simulink model "NeuromuscularModel"  (R2019b)
settings: Solver=ode15s  StartTime=0.0  StopTime=inf  MaxStep=.01  RelTol=1e-4  AbsTol=1e-6  EnableMultiTasking=on
values from neighbouring files (symbols this model uses):
  LceOffsetTA = 1-0.5*w    [ControlParams2.m]
  legLengthClr = .9    (= 0.9)    [ControlParams2.m]    (also in assignGains.m = Gains(20); assignGains2.m = Gains(20); assignGainsSagittal.m = GainsSagittal(39))
  LongDelay = 0.020    (= 0.02)    [ControlParams2.m]
  MidDelay = 0.010    (= 0.01)    [ControlParams2.m]
  N = 82    [vcmaes_1.5cm_0.9ms_Umb10_kneelim1_mstoptorque2.mat]
  ShortDelay = 0.005    [ControlParams2.m]
  simbiconGainD = 5*pi/180    (= 0.0872664625997)    [ControlParams2.m]    (also in assignGains.m = Gains(21); assignGains2.m = Gains(21); assignGainsSagittal.m = GainsSagittal(41))
  simbiconGainDAbd = 0.1421    [ControlParams2.m]    (also in assignGains.m = Gains(33))
  simbiconGainV = 5*pi/180    (= 0.0872664625997)    [ControlParams2.m]    (also in assignGains.m = Gains(22); assignGains2.m = Gains(22); assignGainsSagittal.m = GainsSagittal(42))
  simbiconGainVAbd = 0.2148    [ControlParams2.m]    (also in assignGains.m = Gains(34))
  simbiconLegAngle0 = 85*pi/180    (= 1.4835298642)    [ControlParams2.m]    (also in assignGains.m = Gains(23); assignGains2.m = Gains(23); assignGainsSagittal.m = GainsSagittal(40))
  simbiconLegAngle0Abd = -0.0133    [ControlParams2.m]    (also in assignGains.m = Gains(32))
undefined symbols (not defined in the file or in its folder): footCenterToCGDist, footInertia, footMass, g, hatHipToCenterDistLen, loptGAS, loptTA, lslackGAS, magnitude, phimaxGASa, phimaxGASk, phirefGASa, phirefGASk, rGASa, rGASk, rhoGASa, rhoGASk, X, Y, Z
libraries: NeuroMuscularLibrary x101, nesl_utility x30, sm_lib x21, simulink x4, simulink_extras x2, NeuroMuscularLibrary2 x2
(part 1 of 3)
settings Model: SimulationMode=rapid-accelerator  ParamWorkspaceSource=ReferencedWorkspace  ExtModeTrigDuration=100  TunableVars=GainGAS,GainGLU,GainHAM,GainKneeOverExt,GainSOL,GainSOLTA,GainTA,GainVAS,Kglu,PosGainGG,SpeedGainGG,groundTheta,groundX,groundZ,hipDGain,hipPGain,kneeExtendGain,kneeFlexGain,kneeHoldGain1,kneeHoldGain2,kneeStopGain,legAngleFilter,legLengthClr,simbiconGainD,simbiconGainV,simbiconLegAngle0  TunableVarsStorageClass=Auto,Auto,Auto,Auto,Auto,Auto,Auto,Auto,Auto,Auto,Auto,Auto,Auto,Auto,Auto,Auto,Auto,Auto,Auto,Auto,Auto,Auto,Auto,Auto,Auto,Auto  TunableVarsTypeQualifier=,,,,,,,,,,,,,,,,,,,,,,,,,  Creator=nitisht  LastModifiedBy=Nathan
settings SolverCC: AutoScaleAbsTol=off  ZeroCrossAlgorithm=Adaptive
settings DataIOCC: LimitDataPoints=on  SaveFinalState=on  SaveFormat=StructureWithTime  SaveOutput=off  SaveState=on  ReturnWorkspaceOutputs=off  StateSaveName=tmp_raccel_xout  SignalLoggingName=tmp_raccel_logsout
settings OptimizationCC: DefaultParameterBehavior=Inlined  EfficientMapNaN2IntZero=off  LifeSpan=inf  SimCompilerOptimization=on  AccelVerboseBuild=on
settings DebuggingCC: SaveWithDisabledLinksMsg=none  UnderspecifiedInitializationDetection=Classic  MergeDetectMultiDrivingBlocksExec=none  IgnoredZcDiagnostic=none  SolverPrmCheckMsg=warning  StateNameClashWarn=warning  SFUnexpectedBacktrackingDiag=warning  SFNoUnconditionalDefaultTransitionDiag=warning  SFExecutionAtInitializationDiag=none  ArithmeticOperatorsInVariantConditions=warning
settings HardwareCC: ProdBitPerPointer=32  ProdBitPerSizeT=32  ProdBitPerPtrDiffT=32  ProdLargestAtomicFloat=None  ProdIntDivRoundTo=Undefined  ProdEndianess=Unspecified  ProdWordSize=32  ProdHWDeviceType=Generic->Unspecified (assume 32-bit Generic)  TargetBitPerPointer=64  TargetBitPerSizeT=64  TargetBitPerPtrDiffT=64  TargetLongLongMode=on  TargetIntDivRoundTo=Zero  TargetEndianess=LittleEndian  TargetWordSize=64  TargetHWDeviceType=MATLAB Host  ProdEqTarget=off
settings ModelReferenceCC: PropagateSignalLabelsOutOfModel=off
settings SFSimCC: SFSimEcho=off  SimUseLocalCustomCode=off  CustomCodeUndefinedFunction=UseInterfaceOnly
settings RTWCC: SystemTargetFile=raccel.tlc  TemplateMakefile=raccel_default_tmf  RTWUseLocalCustomCode=off  RTWUseSimCustomCode=on
settings CodeAppCC: GenerateComments=off  MaxIdLength=128  MangleLength=10  SimulinkBlockComments=off
settings RaccelTargetCC: GeneratePreprocessorConditionals=Disable all  MultiInstanceERTCode=off  PreserveStateflowLocalDataDimensions=off  ENABLE_SLEXEC_SSBRIDGE=0  RTWCAPIParams=off
settings ConfigComp: CovMetricSettings=dw  CovHtmlReporting=on  CovSaveCumulativeToWorkspaceVar=on  CovSaveSingleToWorkspaceVar=on  CovExternalEMLEnable=off  CovSFcnEnable=off
settings SimscapeCC: SimscapeNormalizeSystem=off
settings ConfigurationSet: Description=SimMechanics 2G

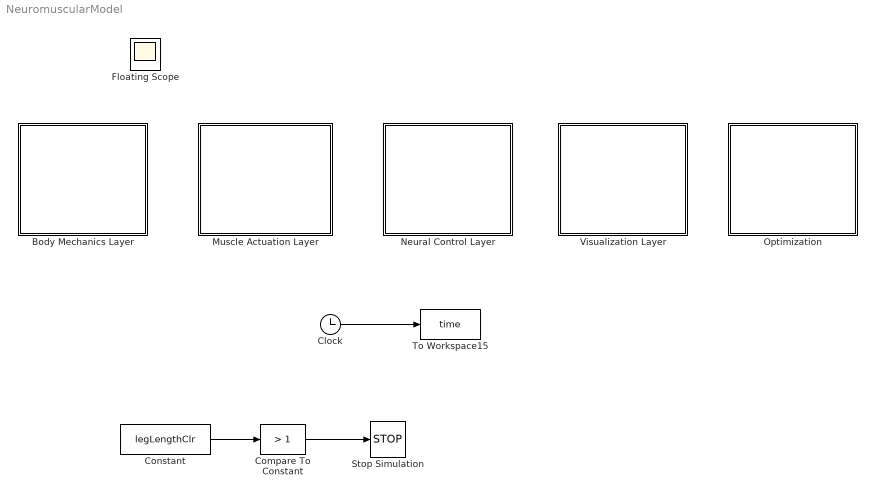
== system NeuromuscularModel ==
  Body Mechanics Layer : Subsystem
  Clock : Clock
  Compare To Constant : simulink/Logic and Bit Operations/Compare To Constant  relop=>  const=1  OutDataTypeStr=boolean
  Constant : Constant  Value=legLengthClr
  Muscle Actuation Layer : Subsystem
  Neural Control Layer : Subsystem
  Optimization : Subsystem
  Stop Simulation : Stop
  To Workspace15 : ToWorkspace  VariableName=time  SampleTime=-1
      settings: MaxDataPoints=1
  Visualization Layer : Subsystem
  Floating Scope : Scope
  wires:
  Clock/1 -> To Workspace15/1
  Compare To Constant/1 -> Stop Simulation/1
  Constant/1 -> Compare To Constant/1

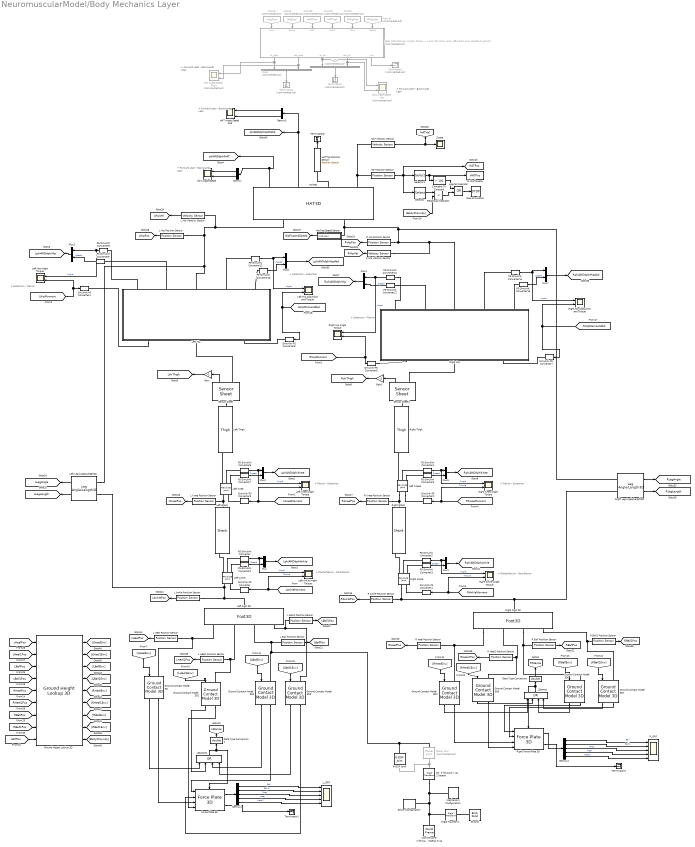
== system NeuromuscularModel/Body Mechanics Layer ==
  note: + Plantarflexion
      | -  Dorsiflexion
  note: + Flexion
      | -  Extension
  note: + Extension
      | -  Flexion
  note: + Forward Lean
      | -  Backwards Lean
  note: + Extension
      | -  Flexion
  note: + Plantarflexion
      | -  Dorsiflexion
  note: + Flexion
      | -  Extension
  note: + Forward Lean
      | -  Backwards Lean
  note: + Abduction
      | -  Adduction
  note: + Forward Lean
      | -  Backwards Lean
  note: + Forward Lean
      | -  Backwards Lean
  6-DOF Joint : sm_lib/Joints/6-DOF Joint  JointMode=Normal  SenseConstraintForce=off  SenseConstraintForceX=off  SenseConstraintForceY=off  SenseConstraintForceZ=off  SenseConstraintTorque=off  SenseConstraintTorqueX=off  SenseConstraintTorqueY=off  SenseConstraintTorqueZ=off  SenseTotalForce=off  SenseTotalForceX=off  SenseTotalForceY=off  SenseTotalForceZ=off  SenseTotalTorque=off  SenseTotalTorqueX=off  SenseTotalTorqueY=off  SenseTotalTorqueZ=off  CompositeWrenchDir=FollowerOnBase  CompositeWrenchFrame=BaseFrame  PxEquilibriumPosition=0  PxEquilibriumPositionUnits=m  PxSpringStiffness=0  PxSpringStiffnessUnits=N/m  PxDampingCoefficient=0  PxDampingCoefficientUnits=N/(m/s)  PxTorqueActuationMode=NoTorque  PxMotionActuationMode=ComputedMotion  PxSensePosition=off  PxSenseVelocity=off  PxSenseAcceleration=off  PxSenseTorqueForce=off  PxSenseLowerLimitTorqueForce=off  PxSenseUpperLimitTorqueForce=off  PxLowerLimitSpecify=off  PxLowerLimitBound=-1  PxLowerLimitBoundUnits=m  PxLowerLimitStiffness=1e6  PxLowerLimitStiffnessUnits=N/m  PxLowerLimitDamping=1e3  PxLowerLimitDampingUnits=N/(m/s)  PxLowerLimitTransitionRegionWidth=1e-4  PxLowerLimitTransitionRegionWidthUnits=m  PxUpperLimitSpecify=off  PxUpperLimitBound=1  PxUpperLimitBoundUnits=m  PxUpperLimitStiffness=1e6  PxUpperLimitStiffnessUnits=N/m  PxUpperLimitDamping=1e3  PxUpperLimitDampingUnits=N/(m/s)  PxUpperLimitTransitionRegionWidth=1e-4  PxUpperLimitTransitionRegionWidthUnits=m  PxPositionTargetSpecify=on  PxPositionTargetPriority=Low  PxPositionTargetValue=0  PxPositionTargetValueUnits=m  PxVelocityTargetSpecify=on  PxVelocityTargetPriority=High  PxVelocityTargetValue=vx0  PxVelocityTargetValueUnits=m/s  PyEquilibriumPosition=0  PyEquilibriumPositionUnits=m  PySpringStiffness=0  PySpringStiffnessUnits=N/m  PyDampingCoefficient=0  PyDampingCoefficientUnits=N/(m/s)  PyTorqueActuationMode=NoTorque  PyMotionActuationMode=ComputedMotion  PySensePosition=off  PySenseVelocity=off  PySenseAcceleration=off  PySenseTorqueForce=off  PySenseLowerLimitTorqueForce=off  PySenseUpperLimitTorqueForce=off  PyLowerLimitSpecify=off  PyLowerLimitBound=-1  PyLowerLimitBoundUnits=m  PyLowerLimitStiffness=1e6  PyLowerLimitStiffnessUnits=N/m  PyLowerLimitDamping=1e3  PyLowerLimitDampingUnits=N/(m/s)  PyLowerLimitTransitionRegionWidth=1e-4  PyLowerLimitTransitionRegionWidthUnits=m  PyUpperLimitSpecify=off  PyUpperLimitBound=1  PyUpperLimitBoundUnits=m  PyUpperLimitStiffness=1e6  PyUpperLimitStiffnessUnits=N/m  PyUpperLimitDamping=1e3  PyUpperLimitDampingUnits=N/(m/s)  PyUpperLimitTransitionRegionWidth=1e-4  PyUpperLimitTransitionRegionWidthUnits=m  PyPositionTargetSpecify=on  PyPositionTargetPriority=Low  PyPositionTargetValue=0  PyPositionTargetValueUnits=m  PyVelocityTargetSpecify=on  PyVelocityTargetPriority=Low  PyVelocityTargetValue=0  PyVelocityTargetValueUnits=m/s  PzEquilibriumPosition=0  PzEquilibriumPositionUnits=m  PzSpringStiffness=0  PzSpringStiffnessUnits=N/m  PzDampingCoefficient=0  PzDampingCoefficientUnits=N/(m/s)  PzTorqueActuationMode=NoTorque  PzMotionActuationMode=ComputedMotion  PzSensePosition=off  PzSenseVelocity=off  PzSenseAcceleration=off  PzSenseTorqueForce=off  PzSenseLowerLimitTorqueForce=off  PzSenseUpperLimitTorqueForce=off  PzLowerLimitSpecify=off  PzLowerLimitBound=-1  PzLowerLimitBoundUnits=m  PzLowerLimitStiffness=1e6  PzLowerLimitStiffnessUnits=N/m  PzLowerLimitDamping=1e3  PzLowerLimitDampingUnits=N/(m/s)  PzLowerLimitTransitionRegionWidth=1e-4  PzLowerLimitTransitionRegionWidthUnits=m  PzUpperLimitSpecify=off  PzUpperLimitBound=1  PzUpperLimitBoundUnits=m  PzUpperLimitStiffness=1e6  PzUpperLimitStiffnessUnits=N/m  PzUpperLimitDamping=1e3  PzUpperLimitDampingUnits=N/(m/s)  PzUpperLimitTransitionRegionWidth=1e-4  PzUpperLimitTransitionRegionWidthUnits=m  PzPositionTargetSpecify=on  PzPositionTargetPriority=Low  PzPositionTargetValue=0  PzPositionTargetValueUnits=m  PzVelocityTargetSpecify=on  PzVelocityTargetPriority=Low  PzVelocityTargetValue=0  PzVelocityTargetValueUnits=m/s  SphDefPosRotationMethod=None  SphDefPosRotationAngleUnits=deg  SphDefPosRotationStandardAxis=+Z  SphDefPosRotationAngle=0.0  SphDefPosRotationArbitraryAxis=[0 0 1]  SphDefPosFollAlignAxisA=+X  SphDefPosBaseAlignAxisA=+Y  SphDefPosFollAlignAxisB=+Y  SphDefPosBaseAlignAxisB=+Z  SphDefPosRotationSequenceAxes=FollowerAxes  SphDefPosRotationSequence=XYX  SphDefPosRotationSequenceAngles=[0 0 0]  SphDefPosRotationSequenceAnglesUnits=deg  SphDefPosRotationMatrix=[1 0 0; 0 1 0; 0 0 1]  SphEqPosRotationMethod=None  SphEqPosRotationAngleUnits=deg  SphEqPosRotationStandardAxis=+Z  SphEqPosRotationAngle=0.0  SphEqPosRotationArbitraryAxis=[0 0 1]  SphEqPosFollAlignAxisA=+X  SphEqPosBaseAlignAxisA=+Y  SphEqPosFollAlignAxisB=+Y  SphEqPosBaseAlignAxisB=+Z  SphEqPosRotationSequenceAxes=FollowerAxes  SphEqPosRotationSequence=XYX  SphEqPosRotationSequenceAngles=[0 0 0]  SphEqPosRotationSequenceAnglesUnits=deg  SphEqPosRotationMatrix=[1 0 0; 0 1 0; 0 0 1]  SphSpringStiffness=0  SphSpringStiffnessUnits=N*m/deg  SphDampingCoefficient=0  SphDampingCoefficientUnits=N*m/(deg/s)  SphActuateTorqueX=off  SphActuateTorqueY=off  SphActuateTorqueZ=off  SphActuateTorque=off  SphTorqueActuationMode=NoTorque  SphMotionActuationMode=ComputedMotion  SphActuationFrame=BaseFrame  SphSensePosition=off  SphSenseVelocityX=off  SphSenseVelocityY=off  SphSenseVelocityZ=off  SphSenseVelocity=off  SphSenseAccelerationX=off  SphSenseAccelerationY=off  SphSenseAccelerationZ=off  SphSenseAcceleration=off  SphSenseTorqueX=off  SphSenseTorqueY=off  SphSenseTorqueZ=off  SphSenseTorqueForce=off  SphSenseLowerLimitTorqueMag=off  SphSenseUpperLimitTorqueMag=off  SphSensingFrame=BaseFrame  SphLowerLimitSpecify=off  SphLowerLimitBound=15  SphLowerLimitBoundUnits=deg  SphLowerLimitStiffness=1e4  SphLowerLimitStiffnessUnits=N*m/deg  SphLowerLimitDamping=10  SphLowerLimitDampingUnits=N*m/(deg/s)  SphLowerLimitTransitionRegionWidth=0.1  SphLowerLimitTransitionRegionWidthUnits=deg  SphUpperLimitSpecify=off  SphUpperLimitBound=45  SphUpperLimitBoundUnits=deg  SphUpperLimitStiffness=1e4  SphUpperLimitStiffnessUnits=N*m/deg  SphUpperLimitDamping=10  SphUpperLimitDampingUnits=N*m/(deg/s)  SphUpperLimitTransitionRegionWidth=0.1  SphUpperLimitTransitionRegionWidthUnits=deg  SphPositionTargetRotationMethod=None  SphPositionTargetRotationAngleUnits=deg  SphPositionTargetRotationStandardAxis=+Z  SphPositionTargetRotationAngle=0.0  SphPositionTargetRotationArbitraryAxis=[0 0 1]  SphPositionTargetFollAlignAxisA=+X  SphPositionTargetBaseAlignAxisA=+Y  SphPositionTargetFollAlignAxisB=+Y  SphPositionTargetBaseAlignAxisB=+Z  SphPositionTargetRotationSequenceAxes=FollowerAxes  SphPositionTargetRotationSequence=XYX  SphPositionTargetRotationSequenceAngles=[0 0 0]  SphPositionTargetRotationSequenceAnglesUnits=deg  SphPositionTargetRotationMatrix=[1 0 0; 0 1 0; 0 0 1]  SphPositionTargetSpecify=on  SphPositionTargetPriority=Low  SphVelocityTargetValue=[0 0 0]  SphVelocityTargetValueUnits=deg/s  SphVelocityTargetSpecify=on  SphVelocityTargetPriority=Low  SphVelocityTargetInFollowerFrame=on
  Compare To Constant : simulink/Logic and Bit Operations/Compare To Constant  relop=>  const=100  OutDataTypeStr=boolean
  Data Type Conversion : DataTypeConversion  OutDataTypeStr=double
  Data Type Conversion1 : DataTypeConversion  OutDataTypeStr=double
  Demux : Demux  Outputs=2
  Demux1 : Demux  Outputs=5
  Demux3 : Demux  Outputs=2
  Demux4 : Demux  Outputs=5
  Force Plate 3D : NeuroMuscularLibrary/Force Plate 3D  SystemSampleTime=-1  Latency=0  AutoFrameSizeCalculation=off
  From10 : From  Commented=on  GotoTag=RHipVel  TagVisibility=global
  From31 : From  Commented=on  GotoTag=HATVel  TagVisibility=global
  From32 : From  Commented=on  GotoTag=HATPos  TagVisibility=global
  From6 : From  Commented=on  GotoTag=LHipVel  TagVisibility=global
  From8 : From  Commented=on  GotoTag=LHipPos  TagVisibility=global
  From9 : From  Commented=on  GotoTag=RHipPos  TagVisibility=global
  Gain : Gain  Gain=-1
  Gain1 : Gain  Gain=-1
  Ground : sm_lib/Body Elements/Brick Solid  GraphicAmbientColor=[0.15 0.15 0.15 1.0]  BasedOnType=Density  BrickDimensions=[3 1 .01]  BrickDimensionUnits=m  CenterOfMass=[-footCenterToCGDist 0 0]  CenterOfMassUnits=m  GraphicDiffuseColor=[0.4 0.2 0.0]  Density=1000  DensityUnits=kg/(m^3)  DoExposeReferenceFrame=on  GraphicEmissiveColor=[0.0 0.0 0.0 1.0]  ExportEntireGeometry=off  SerializedFrames=<Frames/>  MarkerShape=Sphere  MarkerSize=10  GraphicType=FromGeometry  InertiaType=CalculateFromGeometry  Mass=footMass  MassUnits=kg  MomentsOfInertia=[0 0 footInertia]  MomentsOfInertiaUnits=kg*m^2  GraphicOpacity=1.0  ProductsOfInertia=[0 0 0]  ProductsOfInertiaUnits=kg*m^2  GraphicShininess=75  GraphicSpecularColor=[0.5 0.5 0.5 1.0]  GraphicVisPropType=SimpleVisualProperties
  Ground Contact Model 3D{,1..7} (8 alike) : NeuroMuscularLibrary/Ground Contact Model 3D  SystemSampleTime=-1  Latency=0  AutoFrameSizeCalculation=off
  Ground Height Lookup 3D : NeuroMuscularLibrary/Ground Height Lookup 3D  SystemSampleTime=-1  Latency=0  AutoFrameSizeCalculation=off
  HAT Position Sensor : NeuroMuscularLibrary/Position Sensor  SystemSampleTime=-1  Latency=0  AutoFrameSizeCalculation=off
  HAT Angle Speed : Scope  NumInputPorts=2
  HAT Angle Speed Abd : Scope  NumInputPorts=2
  HAT Angle Speed Pitch : Scope  Commented=on  NumInputPorts=2
  HAT Angle Speed Yaw : Scope  Commented=on  NumInputPorts=2
  HAT Velocity Sensor : NeuroMuscularLibrary/Velocity Sensor  SystemSampleTime=-1  Latency=0  AutoFrameSizeCalculation=off
  HAT3D : NeuroMuscularLibrary/HAT3D  SystemSampleTime=-1  Latency=0  AutoFrameSizeCalculation=off
  HATTop Position Sensor : NeuroMuscularLibrary/Position Sensor  SystemSampleTime=-1  Latency=0  AutoFrameSizeCalculation=off
  Hip Pos/Speed Sensor : Subsystem
  L Ankle Position Sensor : NeuroMuscularLibrary/Position Sensor  SystemSampleTime=-1  Latency=0  AutoFrameSizeCalculation=off
  L Ball Position Sensor : NeuroMuscularLibrary/Position Sensor  SystemSampleTime=-1  Latency=0  AutoFrameSizeCalculation=off
  L Ball1 Position Sensor : NeuroMuscularLibrary/Position Sensor  SystemSampleTime=-1  Latency=0  AutoFrameSizeCalculation=off
  L Heel Position Sensor : NeuroMuscularLibrary/Position Sensor  SystemSampleTime=-1  Latency=0  AutoFrameSizeCalculation=off
  L Heel1 Position Sensor : NeuroMuscularLibrary/Position Sensor  SystemSampleTime=-1  Latency=0  AutoFrameSizeCalculation=off
  L Hip Position Sensor : NeuroMuscularLibrary/Position Sensor  SystemSampleTime=-1  Latency=0  AutoFrameSizeCalculation=off
  L Hip Velocity Sensor : NeuroMuscularLibrary/Velocity Sensor  SystemSampleTime=-1  Latency=0  AutoFrameSizeCalculation=off
  L Knee Position Sensor : NeuroMuscularLibrary/Position Sensor  SystemSampleTime=-1  Latency=0  AutoFrameSizeCalculation=off
  LStance : Logic  Operator=OR  Inputs=4  AllPortsSameDT=off
  LStance1 : Logic  Operator=OR  Inputs=4  AllPortsSameDT=off
  L_GRF : Scope  NumInputPorts=5
  Left Ankle : sm_lib/Joints/Revolute Joint  JointMode=Normal  SenseConstraintForce=off  SenseConstraintForceX=off  SenseConstraintForceY=off  SenseConstraintForceZ=off  SenseConstraintTorque=off  SenseConstraintTorqueX=off  SenseConstraintTorqueY=off  SenseConstraintTorqueZ=off  SenseTotalForce=off  SenseTotalForceX=off  SenseTotalForceY=off  SenseTotalForceZ=off  SenseTotalTorque=off  SenseTotalTorqueX=off  SenseTotalTorqueY=off  SenseTotalTorqueZ=off  CompositeWrenchDir=FollowerOnBase  CompositeWrenchFrame=BaseFrame  EquilibriumPosition=0  EquilibriumPositionUnits=deg  SpringStiffness=0  SpringStiffnessUnits=N*m/deg  DampingCoefficient=0  DampingCoefficientUnits=N*m/(deg/s)  TorqueActuationMode=InputTorque  MotionActuationMode=ComputedMotion  SensePosition=on  SenseVelocity=on  SenseAcceleration=off  SenseTorqueForce=off  SenseLowerLimitTorqueForce=off  SenseUpperLimitTorqueForce=off  LowerLimitSpecify=off  LowerLimitBound=-90  LowerLimitBoundUnits=deg  LowerLimitStiffness=1e4  LowerLimitStiffnessUnits=N*m/deg  LowerLimitDamping=10  LowerLimitDampingUnits=N*m/(deg/s)  LowerLimitTransitionRegionWidth=0.1  LowerLimitTransitionRegionWidthUnits=deg  UpperLimitSpecify=off  UpperLimitBound=90  UpperLimitBoundUnits=deg  UpperLimitStiffness=1e4  UpperLimitStiffnessUnits=N*m/deg  UpperLimitDamping=10  UpperLimitDampingUnits=N*m/(deg/s)  UpperLimitTransitionRegionWidth=0.1  UpperLimitTransitionRegionWidthUnits=deg  PositionTargetSpecify=on  PositionTargetPriority=High  PositionTargetValue=LphiAnkle0  PositionTargetValueUnits=rad  VelocityTargetSpecify=on  VelocityTargetPriority=Low  VelocityTargetValue=0  VelocityTargetValueUnits=rad/s
  Left Ankle Angle Torque : Scope  NumInputPorts=2
  Left Foot 3D : NeuroMuscularLibrary/Foot3D  SystemSampleTime=-1  Latency=0  AutoFrameSizeCalculation=off
  Left Hip : Subsystem
  Left Hip Abduction and Torque : Scope  NumInputPorts=2
  Left Hip Angle Torque : Scope  NumInputPorts=2
  Left Knee : sm_lib/Joints/Revolute Joint  JointMode=Normal  SenseConstraintForce=off  SenseConstraintForceX=off  SenseConstraintForceY=off  SenseConstraintForceZ=off  SenseConstraintTorque=off  SenseConstraintTorqueX=off  SenseConstraintTorqueY=off  SenseConstraintTorqueZ=off  SenseTotalForce=off  SenseTotalForceX=off  SenseTotalForceY=off  SenseTotalForceZ=off  SenseTotalTorque=off  SenseTotalTorqueX=off  SenseTotalTorqueY=off  SenseTotalTorqueZ=off  CompositeWrenchDir=FollowerOnBase  CompositeWrenchFrame=BaseFrame  EquilibriumPosition=0  EquilibriumPositionUnits=deg  SpringStiffness=0  SpringStiffnessUnits=N*m/deg  DampingCoefficient=0  DampingCoefficientUnits=N*m/(deg/s)  TorqueActuationMode=InputTorque  MotionActuationMode=ComputedMotion  SensePosition=on  SenseVelocity=on  SenseAcceleration=off  SenseTorqueForce=off  SenseLowerLimitTorqueForce=off  SenseUpperLimitTorqueForce=off  LowerLimitSpecify=off  LowerLimitBound=-90  LowerLimitBoundUnits=deg  LowerLimitStiffness=1e4  LowerLimitStiffnessUnits=N*m/deg  LowerLimitDamping=10  LowerLimitDampingUnits=N*m/(deg/s)  LowerLimitTransitionRegionWidth=0.1  LowerLimitTransitionRegionWidthUnits=deg  UpperLimitSpecify=off  UpperLimitBound=90  UpperLimitBoundUnits=deg  UpperLimitStiffness=1e4  UpperLimitStiffnessUnits=N*m/deg  UpperLimitDamping=10  UpperLimitDampingUnits=N*m/(deg/s)  UpperLimitTransitionRegionWidth=0.1  UpperLimitTransitionRegionWidthUnits=deg  PositionTargetSpecify=on  PositionTargetPriority=High  PositionTargetValue=LphiKnee0  PositionTargetValueUnits=rad  VelocityTargetSpecify=on  VelocityTargetPriority=Low  VelocityTargetValue=0  VelocityTargetValueUnits=deg/s
  Left Knee Angle Torque : Scope  NumInputPorts=2
  Left Knee1 : sm_lib/Joints/Revolute Joint  JointMode=Normal  SenseConstraintForce=off  SenseConstraintForceX=off  SenseConstraintForceY=off  SenseConstraintForceZ=off  SenseConstraintTorque=off  SenseConstraintTorqueX=off  SenseConstraintTorqueY=off  SenseConstraintTorqueZ=off  SenseTotalForce=off  SenseTotalForceX=off  SenseTotalForceY=off  SenseTotalForceZ=off  SenseTotalTorque=off  SenseTotalTorqueX=off  SenseTotalTorqueY=off  SenseTotalTorqueZ=off  CompositeWrenchDir=FollowerOnBase  CompositeWrenchFrame=BaseFrame  EquilibriumPosition=0  EquilibriumPositionUnits=deg  SpringStiffness=0  SpringStiffnessUnits=N*m/deg  DampingCoefficient=0  DampingCoefficientUnits=N*m/(deg/s)  TorqueActuationMode=InputTorque  MotionActuationMode=ComputedMotion  SensePosition=on  SenseVelocity=on  SenseAcceleration=off  SenseTorqueForce=off  SenseLowerLimitTorqueForce=off  SenseUpperLimitTorqueForce=off  LowerLimitSpecify=off  LowerLimitBound=-90  LowerLimitBoundUnits=deg  LowerLimitStiffness=1e4  LowerLimitStiffnessUnits=N*m/deg  LowerLimitDamping=10  LowerLimitDampingUnits=N*m/(deg/s)  LowerLimitTransitionRegionWidth=0.1  LowerLimitTransitionRegionWidthUnits=deg  UpperLimitSpecify=off  UpperLimitBound=90  UpperLimitBoundUnits=deg  UpperLimitStiffness=1e4  UpperLimitStiffnessUnits=N*m/deg  UpperLimitDamping=10  UpperLimitDampingUnits=N*m/(deg/s)  UpperLimitTransitionRegionWidth=0.1  UpperLimitTransitionRegionWidthUnits=deg  PositionTargetSpecify=on  PositionTargetPriority=High  PositionTargetValue=RphiKnee0  PositionTargetValueUnits=rad  VelocityTargetSpecify=on  VelocityTargetPriority=Low  VelocityTargetValue=0  VelocityTargetValueUnits=deg/s
  Left Leg Angle/Length3D : NeuroMuscularLibrary/Leg Angle//Length3D  SystemSampleTime=-1  Latency=0  AutoFrameSizeCalculation=off
  Left Shank : NeuroMuscularLibrary/Shank  SystemSampleTime=-1  Latency=0  AutoFrameSizeCalculation=off
  Left Thigh : NeuroMuscularLibrary/Thigh  SystemSampleTime=-1  Latency=0  AutoFrameSizeCalculation=off
  Logical Operator : Logic  Operator=OR  AllPortsSameDT=off  OutDataTypeStr=boolean
  Mechanism Configuration : sm_lib/Utilities/Mechanism Configuration  UniformGravity=Constant  GravityVector=[0 0 -g]  GravityUnits=m/s^2  LinearizationDelta=0.001
  Mux{,1..7} (8 alike) : Mux  Inputs=2
  Mux8 : Mux  Commented=on  Inputs=2
  Mux9 : Mux  Commented=on  Inputs=2
  PS-Simulink Converter{,2,4,6,8,10,12,14} (8 alike) : nesl_utility/PS-Simulink Converter  PhysicalDomain=network_engine_domain  SubClassName=ps_output  LeftPortType=input  RightPortType=output  PseudoPeriodic=off  Frequencies=[]  Unit=rad  AffineConversion=off
  PS-Simulink Converter{1,3,5,7,9,11,13,15} (8 alike) : nesl_utility/PS-Simulink Converter  PhysicalDomain=network_engine_domain  SubClassName=ps_output  LeftPortType=input  RightPortType=output  PseudoPeriodic=off  Frequencies=[]  Unit=rad/s  AffineConversion=off
  Planar Joint : sm_lib/Joints/Planar Joint  Commented=on  JointMode=Normal  SenseConstraintForce=off  SenseConstraintForceX=off  SenseConstraintForceY=off  SenseConstraintForceZ=off  SenseConstraintTorque=off  SenseConstraintTorqueX=off  SenseConstraintTorqueY=off  SenseConstraintTorqueZ=off  SenseTotalForce=off  SenseTotalForceX=off  SenseTotalForceY=off  SenseTotalForceZ=off  SenseTotalTorque=off  SenseTotalTorqueX=off  SenseTotalTorqueY=off  SenseTotalTorqueZ=off  CompositeWrenchDir=FollowerOnBase  CompositeWrenchFrame=BaseFrame  PxEquilibriumPosition=0  PxEquilibriumPositionUnits=m  PxSpringStiffness=0  PxSpringStiffnessUnits=N/m  PxDampingCoefficient=0  PxDampingCoefficientUnits=N/(m/s)  PxTorqueActuationMode=NoTorque  PxMotionActuationMode=ComputedMotion  PxSensePosition=off  PxSenseVelocity=off  PxSenseAcceleration=off  PxSenseTorqueForce=off  PxSenseLowerLimitTorqueForce=off  PxSenseUpperLimitTorqueForce=off  PxLowerLimitSpecify=off  PxLowerLimitBound=-1  PxLowerLimitBoundUnits=m  PxLowerLimitStiffness=1e6  PxLowerLimitStiffnessUnits=N/m  PxLowerLimitDamping=1e3  PxLowerLimitDampingUnits=N/(m/s)  PxLowerLimitTransitionRegionWidth=1e-4  PxLowerLimitTransitionRegionWidthUnits=m  PxUpperLimitSpecify=off  PxUpperLimitBound=1  PxUpperLimitBoundUnits=m  PxUpperLimitStiffness=1e6  PxUpperLimitStiffnessUnits=N/m  PxUpperLimitDamping=1e3  PxUpperLimitDampingUnits=N/(m/s)  PxUpperLimitTransitionRegionWidth=1e-4  PxUpperLimitTransitionRegionWidthUnits=m  PxPositionTargetSpecify=on  PxPositionTargetPriority=Low  PxPositionTargetValue=0  PxPositionTargetValueUnits=m  PxVelocityTargetSpecify=on  PxVelocityTargetPriority=High  PxVelocityTargetValue=vx0  PxVelocityTargetValueUnits=m/s  PyEquilibriumPosition=0  PyEquilibriumPositionUnits=m  PySpringStiffness=0  PySpringStiffnessUnits=N/m  PyDampingCoefficient=0  PyDampingCoefficientUnits=N/(m/s)  PyTorqueActuationMode=NoTorque  PyMotionActuationMode=ComputedMotion  PySensePosition=off  PySenseVelocity=off  PySenseAcceleration=off  PySenseTorqueForce=off  PySenseLowerLimitTorqueForce=off  PySenseUpperLimitTorqueForce=off  PyLowerLimitSpecify=off  PyLowerLimitBound=-1  PyLowerLimitBoundUnits=m  PyLowerLimitStiffness=1e6  PyLowerLimitStiffnessUnits=N/m  PyLowerLimitDamping=1e3  PyLowerLimitDampingUnits=N/(m/s)  PyLowerLimitTransitionRegionWidth=1e-4  PyLowerLimitTransitionRegionWidthUnits=m  PyUpperLimitSpecify=off  PyUpperLimitBound=1  PyUpperLimitBoundUnits=m  PyUpperLimitStiffness=1e6  PyUpperLimitStiffnessUnits=N/m  PyUpperLimitDamping=1e3  PyUpperLimitDampingUnits=N/(m/s)  PyUpperLimitTransitionRegionWidth=1e-4  PyUpperLimitTransitionRegionWidthUnits=m  PyPositionTargetSpecify=on  PyPositionTargetPriority=Low  PyPositionTargetValue=0  PyPositionTargetValueUnits=m  PyVelocityTargetSpecify=on  PyVelocityTargetPriority=Low  PyVelocityTargetValue=0  PyVelocityTargetValueUnits=m/s  RzEquilibriumPosition=0  RzEquilibriumPositionUnits=deg  RzSpringStiffness=0  RzSpringStiffnessUnits=N*m/deg  RzDampingCoefficient=0  RzDampingCoefficientUnits=N*m/(deg/s)  RzTorqueActuationMode=NoTorque  RzMotionActuationMode=ComputedMotion  RzSensePosition=off  RzSenseVelocity=off  RzSenseAcceleration=off  RzSenseTorqueForce=off  RzSenseLowerLimitTorqueForce=off  RzSenseUpperLimitTorqueForce=off  RzLowerLimitSpecify=off  RzLowerLimitBound=-90  RzLowerLimitBoundUnits=deg  RzLowerLimitStiffness=1e4  RzLowerLimitStiffnessUnits=N*m/deg  RzLowerLimitDamping=10  RzLowerLimitDampingUnits=N*m/(deg/s)  RzLowerLimitTransitionRegionWidth=0.1  RzLowerLimitTransitionRegionWidthUnits=deg  RzUpperLimitSpecify=off  RzUpperLimitBound=90  RzUpperLimitBoundUnits=deg  RzUpperLimitStiffness=1e4  RzUpperLimitStiffnessUnits=N*m/deg  RzUpperLimitDamping=10  RzUpperLimitDampingUnits=N*m/(deg/s)  RzUpperLimitTransitionRegionWidth=0.1  RzUpperLimitTransitionRegionWidthUnits=deg  RzPositionTargetSpecify=on  RzPositionTargetPriority=Low  RzPositionTargetValue=0  RzPositionTargetValueUnits=deg  RzVelocityTargetSpecify=on  RzVelocityTargetPriority=Low  RzVelocityTargetValue=0  RzVelocityTargetValueUnits=deg/s
  R Ankle Position Sensor : NeuroMuscularLibrary/Position Sensor  SystemSampleTime=-1  Latency=0  AutoFrameSizeCalculation=off
  R Ball Position Sensor : NeuroMuscularLibrary/Position Sensor  SystemSampleTime=-1  Latency=0  AutoFrameSizeCalculation=off
  R Ball1 Position Sensor : NeuroMuscularLibrary/Position Sensor  SystemSampleTime=-1  Latency=0  AutoFrameSizeCalculation=off
  R Heel Position Sensor : NeuroMuscularLibrary/Position Sensor  SystemSampleTime=-1  Latency=0  AutoFrameSizeCalculation=off
  R Heel1 Position Sensor : NeuroMuscularLibrary/Position Sensor  SystemSampleTime=-1  Latency=0  AutoFrameSizeCalculation=off
  R Hip Position Sensor : NeuroMuscularLibrary/Position Sensor  SystemSampleTime=-1  Latency=0  AutoFrameSizeCalculation=off
  R Hip Velocity Sensor : NeuroMuscularLibrary/Velocity Sensor  SystemSampleTime=-1  Latency=0  AutoFrameSizeCalculation=off
  R Knee Position Sensor : NeuroMuscularLibrary/Position Sensor  SystemSampleTime=-1  Latency=0  AutoFrameSizeCalculation=off
  R_GRF : Scope  NumInputPorts=5
  Relational Operator : RelationalOperator  Operator=<  OutDataTypeStr=boolean  RndMeth=Nearest
  Rgiht Ankle Angle Torque : Scope  NumInputPorts=2
  Right Ankle : sm_lib/Joints/Revolute Joint  JointMode=Normal  SenseConstraintForce=off  SenseConstraintForceX=off  SenseConstraintForceY=off  SenseConstraintForceZ=off  SenseConstraintTorque=off  SenseConstraintTorqueX=off  SenseConstraintTorqueY=off  SenseConstraintTorqueZ=off  SenseTotalForce=off  SenseTotalForceX=off  SenseTotalForceY=off  SenseTotalForceZ=off  SenseTotalTorque=off  SenseTotalTorqueX=off  SenseTotalTorqueY=off  SenseTotalTorqueZ=off  CompositeWrenchDir=FollowerOnBase  CompositeWrenchFrame=BaseFrame  EquilibriumPosition=0  EquilibriumPositionUnits=deg  SpringStiffness=0  SpringStiffnessUnits=N*m/deg  DampingCoefficient=0  DampingCoefficientUnits=N*m/(deg/s)  TorqueActuationMode=InputTorque  MotionActuationMode=ComputedMotion  SensePosition=on  SenseVelocity=on  SenseAcceleration=off  SenseTorqueForce=off  SenseLowerLimitTorqueForce=off  SenseUpperLimitTorqueForce=off  LowerLimitSpecify=off  LowerLimitBound=-90  LowerLimitBoundUnits=deg  LowerLimitStiffness=1e4  LowerLimitStiffnessUnits=N*m/deg  LowerLimitDamping=10  LowerLimitDampingUnits=N*m/(deg/s)  LowerLimitTransitionRegionWidth=0.1  LowerLimitTransitionRegionWidthUnits=deg  UpperLimitSpecify=off  UpperLimitBound=90  UpperLimitBoundUnits=deg  UpperLimitStiffness=1e4  UpperLimitStiffnessUnits=N*m/deg  UpperLimitDamping=10  UpperLimitDampingUnits=N*m/(deg/s)  UpperLimitTransitionRegionWidth=0.1  UpperLimitTransitionRegionWidthUnits=deg  PositionTargetSpecify=on  PositionTargetPriority=High  PositionTargetValue=RphiAnkle0  PositionTargetValueUnits=rad  VelocityTargetSpecify=on  VelocityTargetPriority=Low  VelocityTargetValue=0  VelocityTargetValueUnits=rad/s
  Right Foot 3D : NeuroMuscularLibrary/Foot3D  SystemSampleTime=-1  Latency=0  AutoFrameSizeCalculation=off
  Right Force Plate 3D : NeuroMuscularLibrary/Force Plate 3D  SystemSampleTime=-1  Latency=0  AutoFrameSizeCalculation=off
  Right Hip : Subsystem
  Right Hip Abduction and Torque : Scope  NumInputPorts=2
  Right Hip Angle Torque : Scope  NumInputPorts=2
  Right Knee Angle Torque : Scope  NumInputPorts=2
  Right Leg Angle/Length3D : NeuroMuscularLibrary/Leg Angle//Length3D  SystemSampleTime=-1  Latency=0  AutoFrameSizeCalculation=off
  Right Shank : NeuroMuscularLibrary/Shank  SystemSampleTime=-1  Latency=0  AutoFrameSizeCalculation=off
  Right Thigh : NeuroMuscularLibrary/Thigh  SystemSampleTime=-1  Latency=0  AutoFrameSizeCalculation=off
  Rigid Transform : sm_lib/Frames and Transforms/Rigid Transform  TranslationMethod=Cartesian  TranslationStandardOffset=1  TranslationLengthUnit=m  TranslationStandardAxis=+X  TranslationCartesianOffset="[1  0 0]"  TranslationROffset=0  TranslationROffsetUnits=m  TranslationZOffset=0  TranslationZOffsetUnits=m  TranslationThetaOffset=0  TranslationThetaOffsetUnits=deg  RotationMethod=None  RotationAngleUnits=deg  RotationStandardAxis=+Z  RotationAngle=0  RotationArbitraryAxis=[0 0 1]  FollAlignAxisA=+X  BaseAlignAxisA=+Y  FollAlignAxisB=+Y  BaseAlignAxisB=+Z  RotationSequenceAxes=FollowerAxes  RotationSequence=XYX  RotationSequenceAngles=[0 0 0]  RotationSequenceAnglesUnits=deg  RotationMatrix=[1 0 0; 0 1 0; 0 0 1]
  Scope : Scope
  Selector : Selector  InputPortWidth=3  IndexOptions=Index vector (dialog)  Indices=[3]  OutputSizes=1
  Selector1 : Selector  InputPortWidth=3  IndexOptions=Index vector (dialog)  Indices=[1]  OutputSizes=1
  Sensor Sheet : NeuroMuscularLibrary/Sensor Sheet  SystemSampleTime=-1  Latency=0  AutoFrameSizeCalculation=off
  Sensor Sheet1 : NeuroMuscularLibrary/Sensor Sheet  SystemSampleTime=-1  Latency=0  AutoFrameSizeCalculation=off
  Simulink-PS Converter{,1..7} (8 alike) : nesl_utility/Simulink-PS Converter  PhysicalDomain=network_engine_domain  SubClassName=ps_input  LeftPortType=input  RightPortType=output  PseudoPeriodic=off  Frequencies=[]  NoiseDistribution=none  NoiseParameters=[]  Unit=N*m  AffineConversion=off  FilteringAndDerivatives=zero  SimscapeFilterOrder=1  InputFilterTimeConstant=0.001  UdotUserProvided=1
  Solver Configuration : nesl_utility/Solver Configuration  PhysicalDomain=network_engine_domain  SubClassName=solver  LeftPortType=input  RightPortType=generic  Tones=[]  Harmonics=[]  SimulateNoise=off  Profile=off  UseLocalSampling=off  EnableSwitchedLinearOptims=on  FrequencyDomain=off  UseCCode=off  RelTol=0.001  AbsTol=1e-06  MinStep=1e-09  ToWorkspace=off  RevertToSquareIcSolve=off  NumHomotopyIterations=100  PhasorMode=off  PhasorModeNumHarmonics=1  DoDC=off  ResidualTolerance=1e-09  UseLocalSolver=off  LocalSolverChoice=NE_BACKWARD_EULER_ADVANCER  LocalSolverSampleTime=0.001  DoFixedCost=off  MaxNonlinIter=3  MaxModeIter=2  LinearAlgebra=Sparse  EquationFormulation=NE_TIME_EF  DelaysMemoryBudget=1024  AutomaticFiltering=on  FilteringTimeConstant=0.001  PartitionStorageMethod=AS_NEEDED  PartitionMemoryBudget=1024  PartitionMethod=FAST
  Stop Simulation : Stop
  TO: X-forward Y-up Z-lateral : sm_lib/Frames and Transforms/Rigid Transform  TranslationMethod=StandardAxis  TranslationStandardOffset=hatLeftHipToCenterDistWidth  TranslationLengthUnit=m  TranslationStandardAxis=+Z  TranslationCartesianOffset=[0 0 0]  TranslationROffset=0  TranslationROffsetUnits=m  TranslationZOffset=0  TranslationZOffsetUnits=m  TranslationThetaOffset=0  TranslationThetaOffsetUnits=deg  RotationMethod=AlignedAxes  RotationAngleUnits=deg  RotationStandardAxis=+Z  RotationAngle=0  RotationArbitraryAxis=[0 0 1]  FollAlignAxisA=+Z  BaseAlignAxisA=+Y  FollAlignAxisB=+X  BaseAlignAxisB=+X  RotationSequenceAxes=FollowerAxes  RotationSequence=XYX  RotationSequenceAngles=[0 0 0]  RotationSequenceAnglesUnits=deg  RotationMatrix=[1 0 0; 0 1 0; 0 0 1]
  Terminator1 : Terminator
  Terminator2 : Terminator  Commented=on
  Terminator3 : Terminator
  Terminator4 : Terminator  Commented=on
  Terminator5 : Terminator  Commented=on
  Terminator6 : Terminator
  To Workspace : ToWorkspace  VariableName=HATPos  SampleTime=-1
      settings: MaxDataPoints=1
  World Frame X-forward Y-lateral Z-up : sm_lib/Frames and Transforms/World Frame
  body pitch/roll/yaw in body frame --- x-axis: forward y-axis: leftward z-axis: parallel to gravity : Subsystem  Commented=on
  tag scope: HATPos=global, HATVel=global, HipPosAndSpeed=global, LAnklePos=global, LBall1Pos=global, LBallPos=global, LHeel1Pos=global, LHeelPos=global, LHipPos=global, LHipVel=global, LKneePos=global, LLegAngle=global, LLegLength=global, LStance=global, LdxThigh=global, LphiANDdphiAnkle=global, LphiANDdphiHip=global, LphiANDdphiHipAbd=global, LphiANDdphiKnee=global, RAnklePos=global, RBall1Pos=global, RBallPos=global, RHeel1Pos=global, RHeelPos=global, RHipPos=global, RHipVel=global, RKneePos=global, RLegAngle=global, RLegLength=global, RStance=global, RdxThigh=global, RphiANDdphiAnkle=global, RphiANDdphiHip=global, RphiANDdphiHipAbd=global, RphiANDdphiKnee=global, phiANDdphiHAT=global, phiANDdphiHATAbd=global
  wires:
  Force Plate 3D/1 -> Demux1/1
  Demux1/1 -> L_GRF/1  "Ball"
  Demux1/2 -> L_GRF/2  "Ball1"
  Demux1/3 -> L_GRF/3  "Total"
  Force Plate 3D/2 -> Terminator1/1
  Ground Contact Model 3D2/2 -> Force Plate 3D/1
  Ground Contact Model 3D/2 -> Force Plate 3D/3
  Ground Contact Model 3D5/2 -> Right Force Plate 3D/1
  Ground Contact Model 3D4/2 -> Right Force Plate 3D/3
  LStance/1 -> Right Force Plate 3D/Enable, Data Type Conversion/1
  Mux/1 -> [LphiANDdphiAnkle]
  [LAnkleMoment] -> Simulink-PS Converter/1, Left Ankle Angle Torque/2  "Torque"
  PS-Simulink Converter6/1 -> Left Knee Angle Torque/1, Mux2/1  "Angle"
  PS-Simulink Converter7/1 -> Mux2/2  "Speed"
  Demux/1 -> HAT Angle Speed/1
  PS-Simulink Converter/1 -> Left Ankle Angle Torque/1, Mux/1  "Angle"
  PS-Simulink Converter1/1 -> Mux/2  "Speed"
  Mux2/1 -> [LphiANDdphiKnee]
  [LKneeMoment] -> Simulink-PS Converter3/1, Left Knee Angle Torque/2
  Sensor Sheet/1 -> Gain/1
  PS-Simulink Converter8/1 -> Mux3/1, Left Hip Angle Torque/1  "Angle"
  PS-Simulink Converter9/1 -> Mux3/2  "Speed"
  HAT3D/1 -> Demux/1, [phiANDdphiHAT]
  Demux/2 -> HAT Angle Speed/2
  Mux3/1 -> [LphiANDdphiHip]
  [LHipMoment] -> Left Hip Angle Torque/2, Simulink-PS Converter4/1
  Gain/1 -> [LdxThigh]
  Sensor Sheet1/1 -> Gain1/1
  Gain1/1 -> [RdxThigh]
  Ground Contact Model 3D4/1 -> LStance/1
  Ground Contact Model 3D5/1 -> LStance/3
  LStance1/1 -> Force Plate 3D/Enable, Data Type Conversion1/1
  Ground Contact Model 3D/1 -> LStance1/1
  Ground Contact Model 3D2/1 -> LStance1/3
  PS-Simulink Converter10/1 -> Right Hip Angle Torque/1, Mux4/1  "Angle"
  PS-Simulink Converter11/1 -> Mux4/2  "Speed"
  [RHipMoment] -> Right Hip Angle Torque/2, Simulink-PS Converter5/1
  Mux5/1 -> [RphiANDdphiKnee]
  Mux1/1 -> [RphiANDdphiAnkle]
  [RAnkleMoment] -> Rgiht Ankle Angle Torque/2, Simulink-PS Converter1/1  "Torque"
  PS-Simulink Converter2/1 -> Rgiht Ankle Angle Torque/1, Mux1/1  "Angle"
  PS-Simulink Converter3/1 -> Mux1/2  "Speed"
  Mux4/1 -> [RphiANDdphiHip]
  L Ankle Position Sensor/1 -> [LAnklePos]
  L Heel Position Sensor/1 -> [LHeelPos]
  R Heel Position Sensor/1 -> [RHeelPos]
  L Knee Position Sensor/1 -> [LKneePos]
  L Hip Position Sensor/1 -> [LHipPos]
  R Hip Position Sensor/1 -> [RHipPos]
  L Ball Position Sensor/1 -> [LBallPos]
  R Ball Position Sensor/1 -> [RBallPos]
  [RKneeMoment] -> Simulink-PS Converter2/1, Right Knee Angle Torque/2  "Torque"
  PS-Simulink Converter4/1 -> Right Knee Angle Torque/1, Mux5/1  "Angle"
  PS-Simulink Converter5/1 -> Mux5/2  "Speed"
  Right Leg Angle/Length3D/1 -> [RLegAngle]
  Right Leg Angle/Length3D/2 -> [RLegLength]
  Left Leg Angle/Length3D/2 -> [LLegLength]
  Left Leg Angle/Length3D/1 -> [LLegAngle]
  Hip Pos/Speed Sensor/1(PosSpeed) -> [HipPosAndSpeed]
  Data Type Conversion/1 -> [RStance]
  Data Type Conversion1/1 -> [LStance]
  [LHeelEnv] -> Ground Contact Model 3D/1
  [LBallEnv] -> Ground Contact Model 3D2/1
  [RHeelEnv] -> Ground Contact Model 3D4/1
  [RBallEnv] -> Ground Contact Model 3D5/1
  R Knee Position Sensor/1 -> [RKneePos]
  R Ankle Position Sensor/1 -> [RAnklePos]
  HATTop Position Sensor/1 -> Terminator6/1
  Selector/1 -> Relational Operator/1
  Selector1/1 -> Compare To Constant/1, To Workspace/1
  HAT Position Sensor/1 -> [HATPos], Selector1/1, Selector/1
  Compare To Constant/1 -> Logical Operator/1
  Relational Operator/1 -> Logical Operator/2
  Logical Operator/1 -> Stop Simulation/1
  [BodyGroundy] -> Relational Operator/2
  HAT Velocity Sensor/1 -> [HATVel], Scope/1
  PS-Simulink Converter12/1 -> Mux6/1, Left Hip Abduction and Torque/1  "Angle"
  PS-Simulink Converter13/1 -> Mux6/2  "Speed"
  [LHipMomentAbd] -> Simulink-PS Converter6/1, Left Hip Abduction and Torque/2
  Mux6/1 -> [LphiANDdphiHipAbd]
  HAT3D/2 -> [phiANDdphiHATAbd], Demux3/1
  Demux3/1 -> HAT Angle Speed Abd/1
  Demux3/2 -> HAT Angle Speed Abd/2
  PS-Simulink Converter14/1 -> Mux7/1, Right Hip Abduction and Torque/1  "Angle"
  PS-Simulink Converter15/1 -> Mux7/2  "Speed"
  Mux7/1 -> [RphiANDdphiHipAbd]
  [RHipMomentAbd] -> Right Hip Abduction and Torque/2, Simulink-PS Converter7/1
  L Heel1 Position Sensor/1 -> [LHeel1Pos]
  [LHeel1Env] -> Ground Contact Model 3D1/1
  Ground Contact Model 3D1/1 -> LStance1/2
  Demux1/4 -> L_GRF/4  "Heel"
  Demux1/5 -> L_GRF/5  "Heel1"
  Ground Contact Model 3D1/2 -> Force Plate 3D/4
  L Ball1 Position Sensor/1 -> [LBall1Pos]
  [LBall1Env] -> Ground Contact Model 3D3/1
  Ground Contact Model 3D3/1 -> LStance1/4
  Ground Contact Model 3D3/2 -> Force Plate 3D/2
  R Heel1 Position Sensor/1 -> [RHeel1Pos]
  [RHeel1Env] -> Ground Contact Model 3D6/1
  Right Force Plate 3D/1 -> Demux4/1
  Demux4/3 -> R_GRF/3  "Total"
  Demux4/4 -> R_GRF/4  "Heel"
  Right Force Plate 3D/2 -> Terminator3/1
  Demux4/5 -> R_GRF/5  "Heel1"
  Demux4/1 -> R_GRF/1  "Ball"
  Demux4/2 -> R_GRF/2  "Ball1"
  Ground Contact Model 3D6/2 -> Right Force Plate 3D/4
  Ground Contact Model 3D6/1 -> LStance/2
  R Ball1 Position Sensor/1 -> [RBall1Pos]
  [RBall1Env] -> Ground Contact Model 3D7/1
  Ground Contact Model 3D7/1 -> LStance/4
  Ground Contact Model 3D7/2 -> Right Force Plate 3D/2
  [HATPos] -> Ground Height Lookup 3D/9
  Ground Height Lookup 3D/9 -> [BodyGroundy]
  Ground Height Lookup 3D/7 -> [RBallEnv]
  [RBallPos] -> Ground Height Lookup 3D/7
  [LHeelPos] -> Ground Height Lookup 3D/1
  [LBallPos] -> Ground Height Lookup 3D/3
  [RHeelPos] -> Ground Height Lookup 3D/5
  Ground Height Lookup 3D/1 -> [LHeelEnv]
  Ground Height Lookup 3D/3 -> [LBallEnv]
  Ground Height Lookup 3D/5 -> [RHeelEnv]
  [LBall1Pos] -> Ground Height Lookup 3D/4
  [RHeel1Pos] -> Ground Height Lookup 3D/6
  [RBall1Pos] -> Ground Height Lookup 3D/8
  Ground Height Lookup 3D/2 -> [LHeel1Env]
  Ground Height Lookup 3D/4 -> [LBall1Env]
  Ground Height Lookup 3D/6 -> [RHeel1Env]
  Ground Height Lookup 3D/8 -> [RBall1Env]
  [LHeel1Pos] -> Ground Height Lookup 3D/2
  body pitch/roll/yaw in body frame --- x-axis: forward y-axis: leftward z-axis: parallel to gravity/2(dth_pitch) -> HAT Angle Speed Pitch/2, Mux8/2
  body pitch/roll/yaw in body frame --- x-axis: forward y-axis: leftward z-axis: parallel to gravity/1(th_pitch) -> HAT Angle Speed Pitch/1, Mux8/1
  body pitch/roll/yaw in body frame --- x-axis: forward y-axis: leftward z-axis: parallel to gravity/3(th_roll) -> Mux9/1, HAT Angle Speed Yaw/1
  body pitch/roll/yaw in body frame --- x-axis: forward y-axis: leftward z-axis: parallel to gravity/4(dth_roll) -> HAT Angle Speed Yaw/2, Mux9/2
  body pitch/roll/yaw in body frame --- x-axis: forward y-axis: leftward z-axis: parallel to gravity/5(yaw) -> Terminator2/1
  L Hip Velocity Sensor/1 -> [LHipVel]
  R Hip Velocity Sensor/1 -> [RHipVel]
  From6/1 -> body pitch/roll/yaw in body frame --- x-axis: forward y-axis: leftward z-axis: parallel to gravity/2(dLHip)
  From10/1 -> body pitch/roll/yaw in body frame --- x-axis: forward y-axis: leftward z-axis: parallel to gravity/6(dRHip)
  From9/1 -> body pitch/roll/yaw in body frame --- x-axis: forward y-axis: leftward z-axis: parallel to gravity/5(RHip)
  From8/1 -> body pitch/roll/yaw in body frame --- x-axis: forward y-axis: leftward z-axis: parallel to gravity/1(LHip)
  From32/1 -> body pitch/roll/yaw in body frame --- x-axis: forward y-axis: leftward z-axis: parallel to gravity/3(HAT)
  From31/1 -> body pitch/roll/yaw in body frame --- x-axis: forward y-axis: leftward z-axis: parallel to gravity/4(dHAT)
  Mux8/1 -> Terminator4/1
  Mux9/1 -> Terminator5/1
  connections:
  TO: X-forward Y-up Z-lateral/RConn1 -- Mechanism Configuration/RConn1 -- Rigid Transform/LConn1 -- World Frame X-forward Y-lateral Z-up/RConn1 -- Solver Configuration/RConn1
  Left Ankle/RConn1 -- Left Shank/LConn1
  Left Ankle/RConn2 -- PS-Simulink Converter/LConn1
  Left Ankle/RConn3 -- PS-Simulink Converter1/LConn1
  Left Knee/RConn1 -- Left Thigh/LConn1
  Left Knee1/RConn1 -- Right Thigh/LConn1
  Left Ankle/LConn2 -- Simulink-PS Converter/RConn1
  Right Ankle/LConn2 -- Simulink-PS Converter1/RConn1
  Right Ankle/RConn2 -- PS-Simulink Converter2/LConn1
  Right Ankle/RConn3 -- PS-Simulink Converter3/LConn1
  Simulink-PS Converter3/RConn1 -- Left Knee/LConn2
  Left Knee/RConn2 -- PS-Simulink Converter6/LConn1
  Left Knee/RConn3 -- PS-Simulink Converter7/LConn1
  Rigid Transform/RConn1 -- Ground/RConn1
  Sensor Sheet/LConn1 -- Left Thigh/RConn1
  Right Thigh/RConn1 -- Sensor Sheet1/LConn1
  Right Hip/LConn2 -- Sensor Sheet1/RConn1
  Simulink-PS Converter5/RConn1 -- Right Hip/LConn1
  PS-Simulink Converter11/LConn1 -- Right Hip/RConn2
  PS-Simulink Converter10/LConn1 -- Right Hip/RConn1
  Left Knee1/RConn2 -- PS-Simulink Converter4/LConn1
  Left Knee1/RConn3 -- PS-Simulink Converter5/LConn1
  Left Knee1/LConn2 -- Simulink-PS Converter2/RConn1
  HAT3D/RConn2 -- HAT Velocity Sensor/LConn1 -- HAT Position Sensor/LConn1
  R Ball Position Sensor/LConn1 -- Ground Contact Model 3D5/LConn1 -- Right Foot 3D/LConn3
  R Heel Position Sensor/LConn1 -- Ground Contact Model 3D4/LConn1 -- Right Foot 3D/LConn1
  L Ball Position Sensor/LConn1 -- Left Foot 3D/LConn3 -- 6-DOF Joint/RConn1 -- Planar Joint/RConn1 -- Ground Contact Model 3D2/LConn1
  L Knee Position Sensor/LConn1 -- Left Knee/LConn1 -- Left Shank/RConn1
  L Hip Position Sensor/LConn1 -- L Hip Velocity Sensor/LConn1 -- HAT3D/LConn1 -- Left Leg Angle/Length3D/LConn1 -- Left Hip/RConn3
  R Hip Position Sensor/LConn1 -- R Hip Velocity Sensor/LConn1 -- Right Hip/RConn3 -- Right Leg Angle/Length3D/LConn1 -- Hip Pos/Speed Sensor/LConn1 -- HAT3D/LConn2
  Right Shank/RConn1 -- Left Knee1/LConn1 -- R Knee Position Sensor/LConn1
  Right Ankle/RConn1 -- Right Shank/LConn1
  R Ankle Position Sensor/LConn1 -- Right Ankle/LConn1 -- Right Leg Angle/Length3D/LConn2 -- Right Foot 3D/RConn1
  L Heel Position Sensor/LConn1 -- Ground Contact Model 3D/LConn1 -- Left Foot 3D/LConn1
  Left Leg Angle/Length3D/LConn2 -- Left Ankle/LConn1 -- Left Foot 3D/RConn1 -- L Ankle Position Sensor/LConn1
  Planar Joint/LConn1 -- 6-DOF Joint/LConn1 -- TO: X-forward Y-up Z-lateral/LConn1
  HAT3D/RConn1 -- HATTop Position Sensor/LConn1
  Left Hip/RConn1 -- PS-Simulink Converter8/LConn1
  Left Hip/RConn2 -- PS-Simulink Converter9/LConn1
  Left Hip/LConn1 -- Simulink-PS Converter4/RConn1
  Sensor Sheet/RConn1 -- Left Hip/LConn2
  PS-Simulink Converter12/LConn1 -- Left Hip/RConn4
  Left Hip/RConn5 -- PS-Simulink Converter13/LConn1
  Simulink-PS Converter6/RConn1 -- Left Hip/LConn3
  Right Hip/RConn5 -- PS-Simulink Converter15/LConn1
  Right Hip/RConn4 -- PS-Simulink Converter14/LConn1
  Right Hip/LConn3 -- Simulink-PS Converter7/RConn1
  L Heel1 Position Sensor/LConn1 -- Ground Contact Model 3D1/LConn1 -- Left Foot 3D/LConn2
  Left Foot 3D/LConn4 -- Ground Contact Model 3D3/LConn1 -- L Ball1 Position Sensor/LConn1
  R Heel1 Position Sensor/LConn1 -- Ground Contact Model 3D6/LConn1 -- Right Foot 3D/LConn2
  Right Foot 3D/LConn4 -- Ground Contact Model 3D7/LConn1 -- R Ball1 Position Sensor/LConn1
